simulink model "VCU_CS75_12_16_Test"  (R2014a)
settings: Solver=FixedStepDiscrete  StartTime=0.0  StopTime=25  FixedStep=0.0005  RelTol=1e-3
undefined symbols (not defined in the file): ecucoder_acal, I_SW01_L, LaterlAngleCommand, LDW, RemoteAcclPosition
libraries: simulink x913, ec5744lib x39
(part 23 of 30)

== system VCU_CS75_12_16_Test/长安CS75底盘程序，20ms一次/Output/Subsystem/TransmitMessages5/ACC_3F5/CRC ==
  CRC : Inport
  CRCRon : Rounding  Operator=round
  CRC_1sat : Saturate  UpperLimit=255  LowerLimit=0
  CRC_Convert : DataTypeConversion  OutDataTypeStr=uint8
  CRC_Convert1 : DataTypeConversion  OutDataTypeStr=uint32
  CRC_D : Product  Inputs=*/
  CRC_F : Constant  OutDataTypeStr=single
  CRC_L : simulink/Logic and Bit Operations/Bitwise Operator  logicop=AND  UseBitMask=on  BitMask=255  BitMaskRealWorld=Stored Integer
  CRC_O : Constant  Value=0  OutDataTypeStr=single
  CRC_S : ArithShift
  CRC_sat : Saturate  UpperLimit=0  LowerLimit=0
  CRC_st : Sum  Inputs=+-
  Constant{1..7} (7 alike) : Constant  Value=0  OutDataTypeStr=uint8
  output1 : Outport
  output2 : Outport  Port=2
  output3 : Outport  Port=3
  output4 : Outport  Port=4
  output5 : Outport  Port=5
  output6 : Outport  Port=6
  output7 : Outport  Port=7
  output8 : Outport  Port=8
  wires:
  CRC/1 -> CRC_sat/1
  CRC_sat/1 -> CRC_st/1
  CRC_O/1 -> CRC_st/2
  CRC_st/1 -> CRC_D/1
  CRC_F/1 -> CRC_D/2
  CRC_D/1 -> CRCRon/1
  CRCRon/1 -> CRC_S/1
  CRC_S/1 -> CRC_1sat/1
  CRC_1sat/1 -> CRC_Convert1/1
  CRC_Convert1/1 -> CRC_L/1
  CRC_L/1 -> CRC_Convert/1
  CRC_Convert/1 -> output8/1
  Constant1/1 -> output1/1
  Constant2/1 -> output2/1
  Constant3/1 -> output3/1
  Constant4/1 -> output4/1
  Constant5/1 -> output5/1
  Constant6/1 -> output6/1
  Constant7/1 -> output7/1

== system VCU_CS75_12_16_Test/长安CS75底盘程序，20ms一次/Output/Subsystem/TransmitMessages5/ACC_3F5/RollingConter ==
  RollingConter : Inport
  Constant{1..6,8} (7 alike) : Constant  Value=0  OutDataTypeStr=uint8
  RollingConterRon : Rounding  Operator=round
  RollingConter_1sat : Saturate  UpperLimit=15  LowerLimit=0
  RollingConter_Convert : DataTypeConversion  OutDataTypeStr=uint8
  RollingConter_Convert1 : DataTypeConversion  OutDataTypeStr=uint32
  RollingConter_D : Product  Inputs=*/
  RollingConter_F : Constant  OutDataTypeStr=single
  RollingConter_L : simulink/Logic and Bit Operations/Bitwise Operator  logicop=AND  UseBitMask=on  BitMask=15  BitMaskRealWorld=Stored Integer
  RollingConter_O : Constant  Value=0  OutDataTypeStr=single
  RollingConter_S : ArithShift
  RollingConter_sat : Saturate  UpperLimit=0  LowerLimit=0
  RollingConter_st : Sum  Inputs=+-
  output1 : Outport
  output2 : Outport  Port=2
  output3 : Outport  Port=3
  output4 : Outport  Port=4
  output5 : Outport  Port=5
  output6 : Outport  Port=6
  output7 : Outport  Port=7
  output8 : Outport  Port=8
  wires:
  RollingConter/1 -> RollingConter_sat/1
  RollingConter_sat/1 -> RollingConter_st/1
  RollingConter_O/1 -> RollingConter_st/2
  RollingConter_st/1 -> RollingConter_D/1
  RollingConter_F/1 -> RollingConter_D/2
  RollingConter_D/1 -> RollingConterRon/1
  RollingConterRon/1 -> RollingConter_S/1
  RollingConter_S/1 -> RollingConter_1sat/1
  RollingConter_1sat/1 -> RollingConter_Convert1/1
  RollingConter_Convert1/1 -> RollingConter_L/1
  RollingConter_L/1 -> RollingConter_Convert/1
  RollingConter_Convert/1 -> output7/1
  Constant1/1 -> output1/1
  Constant2/1 -> output2/1
  Constant3/1 -> output3/1
  Constant4/1 -> output4/1
  Constant5/1 -> output5/1
  Constant6/1 -> output6/1
  Constant8/1 -> output8/1

== system VCU_CS75_12_16_Test/长安CS75底盘程序，20ms一次/Output/Subsystem/TransmitMessages7/APA_29A/APA_ActivationStatus ==
  APA_ActivationStatus : Inport
  APA_ActivationStatusRon : Rounding  Operator=round
  APA_ActivationStatus_1sat : Saturate  UpperLimit=224  LowerLimit=0
  APA_ActivationStatus_Convert : DataTypeConversion  OutDataTypeStr=uint8
  APA_ActivationStatus_Convert1 : DataTypeConversion  OutDataTypeStr=uint32
  APA_ActivationStatus_D : Product  Inputs=*/
  APA_ActivationStatus_F : Constant  OutDataTypeStr=single
  APA_ActivationStatus_L : simulink/Logic and Bit Operations/Bitwise Operator  logicop=AND  UseBitMask=on  BitMask=224  BitMaskRealWorld=Stored Integer
  APA_ActivationStatus_O : Constant  Value=0  OutDataTypeStr=single
  APA_ActivationStatus_S : ArithShift  BitShiftNumber=-5
  APA_ActivationStatus_sat : Saturate  UpperLimit=7  LowerLimit=0
  APA_ActivationStatus_st : Sum  Inputs=+-
  Constant{1..5,7..8} (7 alike) : Constant  Value=0  OutDataTypeStr=uint8
  output1 : Outport
  output2 : Outport  Port=2
  output3 : Outport  Port=3
  output4 : Outport  Port=4
  output5 : Outport  Port=5
  output6 : Outport  Port=6
  output7 : Outport  Port=7
  output8 : Outport  Port=8
  wires:
  APA_ActivationStatus/1 -> APA_ActivationStatus_sat/1
  APA_ActivationStatus_sat/1 -> APA_ActivationStatus_st/1
  APA_ActivationStatus_O/1 -> APA_ActivationStatus_st/2
  APA_ActivationStatus_st/1 -> APA_ActivationStatus_D/1
  APA_ActivationStatus_F/1 -> APA_ActivationStatus_D/2
  APA_ActivationStatus_D/1 -> APA_ActivationStatusRon/1
  APA_ActivationStatusRon/1 -> APA_ActivationStatus_S/1
  APA_ActivationStatus_S/1 -> APA_ActivationStatus_1sat/1
  APA_ActivationStatus_1sat/1 -> APA_ActivationStatus_Convert1/1
  APA_ActivationStatus_Convert1/1 -> APA_ActivationStatus_L/1
  APA_ActivationStatus_L/1 -> APA_ActivationStatus_Convert/1
  APA_ActivationStatus_Convert/1 -> output6/1
  Constant1/1 -> output1/1
  Constant2/1 -> output2/1
  Constant3/1 -> output3/1
  Constant4/1 -> output4/1
  Constant5/1 -> output5/1
  Constant7/1 -> output7/1
  Constant8/1 -> output8/1

== system VCU_CS75_12_16_Test/长安CS75底盘程序，20ms一次/Output/Subsystem/TransmitMessages7/APA_29A/APA_Checksum ==
  APA_Checksum : Inport
  APA_ChecksumRon : Rounding  Operator=round
  APA_Checksum_1sat : Saturate  UpperLimit=240  LowerLimit=0
  APA_Checksum_Convert : DataTypeConversion  OutDataTypeStr=uint8
  APA_Checksum_Convert1 : DataTypeConversion  OutDataTypeStr=uint32
  APA_Checksum_D : Product  Inputs=*/
  APA_Checksum_F : Constant  OutDataTypeStr=single
  APA_Checksum_L : simulink/Logic and Bit Operations/Bitwise Operator  logicop=AND  UseBitMask=on  BitMask=240  BitMaskRealWorld=Stored Integer
  APA_Checksum_O : Constant  Value=0  OutDataTypeStr=single
  APA_Checksum_S : ArithShift  BitShiftNumber=-4
  APA_Checksum_sat : Saturate  UpperLimit=0  LowerLimit=0
  APA_Checksum_st : Sum  Inputs=+-
  Constant{1..7} (7 alike) : Constant  Value=0  OutDataTypeStr=uint8
  output1 : Outport
  output2 : Outport  Port=2
  output3 : Outport  Port=3
  output4 : Outport  Port=4
  output5 : Outport  Port=5
  output6 : Outport  Port=6
  output7 : Outport  Port=7
  output8 : Outport  Port=8
  wires:
  APA_Checksum/1 -> APA_Checksum_sat/1
  APA_Checksum_sat/1 -> APA_Checksum_st/1
  APA_Checksum_O/1 -> APA_Checksum_st/2
  APA_Checksum_st/1 -> APA_Checksum_D/1
  APA_Checksum_F/1 -> APA_Checksum_D/2
  APA_Checksum_D/1 -> APA_ChecksumRon/1
  APA_ChecksumRon/1 -> APA_Checksum_S/1
  APA_Checksum_S/1 -> APA_Checksum_1sat/1
  APA_Checksum_1sat/1 -> APA_Checksum_Convert1/1
  APA_Checksum_Convert1/1 -> APA_Checksum_L/1
  APA_Checksum_L/1 -> APA_Checksum_Convert/1
  APA_Checksum_Convert/1 -> output8/1
  Constant1/1 -> output1/1
  Constant2/1 -> output2/1
  Constant3/1 -> output3/1
  Constant4/1 -> output4/1
  Constant5/1 -> output5/1
  Constant6/1 -> output6/1
  Constant7/1 -> output7/1

== system VCU_CS75_12_16_Test/长安CS75底盘程序，20ms一次/Output/Subsystem/TransmitMessages7/APA_29A/APA_EPBrequest ==
  APA_EPBrequest : Inport
  APA_EPBrequestRon : Rounding  Operator=round
  APA_EPBrequest_1sat : Saturate  UpperLimit=3  LowerLimit=0
  APA_EPBrequest_Convert : DataTypeConversion  OutDataTypeStr=uint8
  APA_EPBrequest_Convert1 : DataTypeConversion  OutDataTypeStr=uint32
  APA_EPBrequest_D : Product  Inputs=*/
  APA_EPBrequest_F : Constant  OutDataTypeStr=single
  APA_EPBrequest_L : simulink/Logic and Bit Operations/Bitwise Operator  logicop=AND  UseBitMask=on  BitMask=3  BitMaskRealWorld=Stored Integer
  APA_EPBrequest_O : Constant  Value=0  OutDataTypeStr=single
  APA_EPBrequest_S : ArithShift
  APA_EPBrequest_sat : Saturate  UpperLimit=0  LowerLimit=0
  APA_EPBrequest_st : Sum  Inputs=+-
  Constant{2..8} (7 alike) : Constant  Value=0  OutDataTypeStr=uint8
  output1 : Outport
  output2 : Outport  Port=2
  output3 : Outport  Port=3
  output4 : Outport  Port=4
  output5 : Outport  Port=5
  output6 : Outport  Port=6
  output7 : Outport  Port=7
  output8 : Outport  Port=8
  wires:
  APA_EPBrequest/1 -> APA_EPBrequest_sat/1
  APA_EPBrequest_sat/1 -> APA_EPBrequest_st/1
  APA_EPBrequest_O/1 -> APA_EPBrequest_st/2
  APA_EPBrequest_st/1 -> APA_EPBrequest_D/1
  APA_EPBrequest_F/1 -> APA_EPBrequest_D/2
  APA_EPBrequest_D/1 -> APA_EPBrequestRon/1
  APA_EPBrequestRon/1 -> APA_EPBrequest_S/1
  APA_EPBrequest_S/1 -> APA_EPBrequest_1sat/1
  APA_EPBrequest_1sat/1 -> APA_EPBrequest_Convert1/1
  APA_EPBrequest_Convert1/1 -> APA_EPBrequest_L/1
  APA_EPBrequest_L/1 -> APA_EPBrequest_Convert/1
  APA_EPBrequest_Convert/1 -> output1/1
  Constant2/1 -> output2/1
  Constant3/1 -> output3/1
  Constant4/1 -> output4/1
  Constant5/1 -> output5/1
  Constant6/1 -> output6/1
  Constant7/1 -> output7/1
  Constant8/1 -> output8/1

== system VCU_CS75_12_16_Test/长安CS75底盘程序，20ms一次/Output/Subsystem/TransmitMessages7/APA_29A/APA_EPBrequestValid ==
  APA_EPBrequestValid : Inport
  APA_EPBrequestValidRon : Rounding  Operator=round
  APA_EPBrequestValid_1sat : Saturate  UpperLimit=4  LowerLimit=0
  APA_EPBrequestValid_Convert : DataTypeConversion  OutDataTypeStr=uint8
  APA_EPBrequestValid_Convert1 : DataTypeConversion  OutDataTypeStr=uint32
  APA_EPBrequestValid_D : Product  Inputs=*/
  APA_EPBrequestValid_F : Constant  OutDataTypeStr=single
  APA_EPBrequestValid_L : simulink/Logic and Bit Operations/Bitwise Operator  logicop=AND  UseBitMask=on  BitMask=4  BitMaskRealWorld=Stored Integer
  APA_EPBrequestValid_O : Constant  Value=0  OutDataTypeStr=single
  APA_EPBrequestValid_S : ArithShift  BitShiftNumber=-2
  APA_EPBrequestValid_sat : Saturate  UpperLimit=0  LowerLimit=0
  APA_EPBrequestValid_st : Sum  Inputs=+-
  Constant{2..8} (7 alike) : Constant  Value=0  OutDataTypeStr=uint8
  output1 : Outport
  output2 : Outport  Port=2
  output3 : Outport  Port=3
  output4 : Outport  Port=4
  output5 : Outport  Port=5
  output6 : Outport  Port=6
  output7 : Outport  Port=7
  output8 : Outport  Port=8
  wires:
  APA_EPBrequestValid/1 -> APA_EPBrequestValid_sat/1
  APA_EPBrequestValid_sat/1 -> APA_EPBrequestValid_st/1
  APA_EPBrequestValid_O/1 -> APA_EPBrequestValid_st/2
  APA_EPBrequestValid_st/1 -> APA_EPBrequestValid_D/1
  APA_EPBrequestValid_F/1 -> APA_EPBrequestValid_D/2
  APA_EPBrequestValid_D/1 -> APA_EPBrequestValidRon/1
  APA_EPBrequestValidRon/1 -> APA_EPBrequestValid_S/1
  APA_EPBrequestValid_S/1 -> APA_EPBrequestValid_1sat/1
  APA_EPBrequestValid_1sat/1 -> APA_EPBrequestValid_Convert1/1
  APA_EPBrequestValid_Convert1/1 -> APA_EPBrequestValid_L/1
  APA_EPBrequestValid_L/1 -> APA_EPBrequestValid_Convert/1
  APA_EPBrequestValid_Convert/1 -> output1/1
  Constant2/1 -> output2/1
  Constant3/1 -> output3/1
  Constant4/1 -> output4/1
  Constant5/1 -> output5/1
  Constant6/1 -> output6/1
  Constant7/1 -> output7/1
  Constant8/1 -> output8/1

== system VCU_CS75_12_16_Test/长安CS75底盘程序，20ms一次/Output/Subsystem/TransmitMessages7/APA_29A/APA_GearReqValid ==
  APA_GearReqValid : Inport
  APA_GearReqValidRon : Rounding  Operator=round
  APA_GearReqValid_1sat : Saturate  UpperLimit=4  LowerLimit=0
  APA_GearReqValid_Convert : DataTypeConversion  OutDataTypeStr=uint8
  APA_GearReqValid_Convert1 : DataTypeConversion  OutDataTypeStr=uint32
  APA_GearReqValid_D : Product  Inputs=*/
  APA_GearReqValid_F : Constant  OutDataTypeStr=single
  APA_GearReqValid_L : simulink/Logic and Bit Operations/Bitwise Operator  logicop=AND  UseBitMask=on  BitMask=4  BitMaskRealWorld=Stored Integer
  APA_GearReqValid_O : Constant  Value=0  OutDataTypeStr=single
  APA_GearReqValid_S : ArithShift  BitShiftNumber=-2
  APA_GearReqValid_sat : Saturate  UpperLimit=1  LowerLimit=0
  APA_GearReqValid_st : Sum  Inputs=+-
  Constant{1..3,5..8} (7 alike) : Constant  Value=0  OutDataTypeStr=uint8
  output1 : Outport
  output2 : Outport  Port=2
  output3 : Outport  Port=3
  output4 : Outport  Port=4
  output5 : Outport  Port=5
  output6 : Outport  Port=6
  output7 : Outport  Port=7
  output8 : Outport  Port=8
  wires:
  APA_GearReqValid/1 -> APA_GearReqValid_sat/1
  APA_GearReqValid_sat/1 -> APA_GearReqValid_st/1
  APA_GearReqValid_O/1 -> APA_GearReqValid_st/2
  APA_GearReqValid_st/1 -> APA_GearReqValid_D/1
  APA_GearReqValid_F/1 -> APA_GearReqValid_D/2
  APA_GearReqValid_D/1 -> APA_GearReqValidRon/1
  APA_GearReqValidRon/1 -> APA_GearReqValid_S/1
  APA_GearReqValid_S/1 -> APA_GearReqValid_1sat/1
  APA_GearReqValid_1sat/1 -> APA_GearReqValid_Convert1/1
  APA_GearReqValid_Convert1/1 -> APA_GearReqValid_L/1
  APA_GearReqValid_L/1 -> APA_GearReqValid_Convert/1
  APA_GearReqValid_Convert/1 -> output4/1
  Constant1/1 -> output1/1
  Constant2/1 -> output2/1
  Constant3/1 -> output3/1
  Constant5/1 -> output5/1
  Constant6/1 -> output6/1
  Constant7/1 -> output7/1
  Constant8/1 -> output8/1

== system VCU_CS75_12_16_Test/长安CS75底盘程序，20ms一次/Output/Subsystem/TransmitMessages7/APA_29A/APA_LSCAction ==
  APA_LSCAction : Inport
  APA_LSCActionRon : Rounding  Operator=round
  APA_LSCAction_1sat : Saturate  UpperLimit=8  LowerLimit=0
  APA_LSCAction_Convert : DataTypeConversion  OutDataTypeStr=uint8
  APA_LSCAction_Convert1 : DataTypeConversion  OutDataTypeStr=uint32
  APA_LSCAction_D : Product  Inputs=*/
  APA_LSCAction_F : Constant  OutDataTypeStr=single
  APA_LSCAction_L : simulink/Logic and Bit Operations/Bitwise Operator  logicop=AND  UseBitMask=on  BitMask=8  BitMaskRealWorld=Stored Integer
  APA_LSCAction_O : Constant  Value=0  OutDataTypeStr=single
  APA_LSCAction_S : ArithShift  BitShiftNumber=-3
  APA_LSCAction_sat : Saturate  UpperLimit=0  LowerLimit=0
  APA_LSCAction_st : Sum  Inputs=+-
  Constant{1..3,5..8} (7 alike) : Constant  Value=0  OutDataTypeStr=uint8
  output1 : Outport
  output2 : Outport  Port=2
  output3 : Outport  Port=3
  output4 : Outport  Port=4
  output5 : Outport  Port=5
  output6 : Outport  Port=6
  output7 : Outport  Port=7
  output8 : Outport  Port=8
  wires:
  APA_LSCAction/1 -> APA_LSCAction_sat/1
  APA_LSCAction_sat/1 -> APA_LSCAction_st/1
  APA_LSCAction_O/1 -> APA_LSCAction_st/2
  APA_LSCAction_st/1 -> APA_LSCAction_D/1
  APA_LSCAction_F/1 -> APA_LSCAction_D/2
  APA_LSCAction_D/1 -> APA_LSCActionRon/1
  APA_LSCActionRon/1 -> APA_LSCAction_S/1
  APA_LSCAction_S/1 -> APA_LSCAction_1sat/1
  APA_LSCAction_1sat/1 -> APA_LSCAction_Convert1/1
  APA_LSCAction_Convert1/1 -> APA_LSCAction_L/1
  APA_LSCAction_L/1 -> APA_LSCAction_Convert/1
  APA_LSCAction_Convert/1 -> output4/1
  Constant1/1 -> output1/1
  Constant2/1 -> output2/1
  Constant3/1 -> output3/1
  Constant5/1 -> output5/1
  Constant6/1 -> output6/1
  Constant7/1 -> output7/1
  Constant8/1 -> output8/1

== system VCU_CS75_12_16_Test/长安CS75底盘程序，20ms一次/Output/Subsystem/TransmitMessages7/APA_29A/APA_RollingCounter ==
  APA_RollingCounter : Inport
  APA_RollingCounterRon : Rounding  Operator=round
  APA_RollingCounter_1sat : Saturate  UpperLimit=15  LowerLimit=0
  APA_RollingCounter_Convert : DataTypeConversion  OutDataTypeStr=uint8
  APA_RollingCounter_Convert1 : DataTypeConversion  OutDataTypeStr=uint32
  APA_RollingCounter_D : Product  Inputs=*/
  APA_RollingCounter_F : Constant  OutDataTypeStr=single
  APA_RollingCounter_L : simulink/Logic and Bit Operations/Bitwise Operator  logicop=AND  UseBitMask=on  BitMask=15  BitMaskRealWorld=Stored Integer
  APA_RollingCounter_O : Constant  Value=0  OutDataTypeStr=single
  APA_RollingCounter_S : ArithShift
  APA_RollingCounter_sat : Saturate  UpperLimit=0  LowerLimit=0
  APA_RollingCounter_st : Sum  Inputs=+-
  Constant{1..7} (7 alike) : Constant  Value=0  OutDataTypeStr=uint8
  output1 : Outport
  output2 : Outport  Port=2
  output3 : Outport  Port=3
  output4 : Outport  Port=4
  output5 : Outport  Port=5
  output6 : Outport  Port=6
  output7 : Outport  Port=7
  output8 : Outport  Port=8
  wires:
  APA_RollingCounter/1 -> APA_RollingCounter_sat/1
  APA_RollingCounter_sat/1 -> APA_RollingCounter_st/1
  APA_RollingCounter_O/1 -> APA_RollingCounter_st/2
  APA_RollingCounter_st/1 -> APA_RollingCounter_D/1
  APA_RollingCounter_F/1 -> APA_RollingCounter_D/2
  APA_RollingCounter_D/1 -> APA_RollingCounterRon/1
  APA_RollingCounterRon/1 -> APA_RollingCounter_S/1
  APA_RollingCounter_S/1 -> APA_RollingCounter_1sat/1
  APA_RollingCounter_1sat/1 -> APA_RollingCounter_Convert1/1
  APA_RollingCounter_Convert1/1 -> APA_RollingCounter_L/1
  APA_RollingCounter_L/1 -> APA_RollingCounter_Convert/1
  APA_RollingCounter_Convert/1 -> output8/1
  Constant1/1 -> output1/1
  Constant2/1 -> output2/1
  Constant3/1 -> output3/1
  Constant4/1 -> output4/1
  Constant5/1 -> output5/1
  Constant6/1 -> output6/1
  Constant7/1 -> output7/1

== system VCU_CS75_12_16_Test/长安CS75底盘程序，20ms一次/Output/Subsystem/TransmitMessages7/APA_29A/APA_TargetAcceleration ==
  APA_TargetAcceleration : Inport
  APA_TargetAccelerationBitCov : DataTypeConversion  OutDataTypeStr=uint8
  APA_TargetAccelerationCOV : DataTypeConversion  OutDataTypeStr=uint8
  APA_TargetAccelerationRon : Rounding  Operator=round
  APA_TargetAcceleration_1sat : Saturate  UpperLimit=16320  LowerLimit=0
  APA_TargetAcceleration_And : simulink/Logic and Bit Operations/Bitwise Operator  logicop=AND  UseBitMask=off  NumInputPorts=2  BitMask=bin2dec('11011001')  BitMaskRealWorld=Stored Integer
  APA_TargetAcceleration_And_C : Constant  Value=255  OutDataTypeStr=uint32
  APA_TargetAcceleration_Convert : DataTypeConversion  OutDataTypeStr=uint32
  APA_TargetAcceleration_D : Product  Inputs=*/
  APA_TargetAcceleration_D1 : Product  Inputs=*/
  APA_TargetAcceleration_F : Constant  Value=0.05  OutDataTypeStr=single
  APA_TargetAcceleration_L : simulink/Logic and Bit Operations/Bitwise Operator  logicop=AND  UseBitMask=on  BitMask=16320  BitMaskRealWorld=Stored Integer
  APA_TargetAcceleration_O : Constant  Value=-5  OutDataTypeStr=single
  APA_TargetAcceleration_S : ArithShift  BitShiftNumber=-6
  APA_TargetAcceleration_sat : Saturate  UpperLimit=0  LowerLimit=0
  APA_TargetAcceleration_st : Sum  Inputs=+-
  APA_TargetAccelerationoutput2_C : Constant  Value=256
  Constant{1,4..8} (6 alike) : Constant  Value=0  OutDataTypeStr=uint8
  output1 : Outport
  output2 : Outport  Port=2
  output3 : Outport  Port=3
  output4 : Outport  Port=4
  output5 : Outport  Port=5
  output6 : Outport  Port=6
  output7 : Outport  Port=7
  output8 : Outport  Port=8
  wires:
  APA_TargetAcceleration/1 -> APA_TargetAcceleration_sat/1
  APA_TargetAcceleration_sat/1 -> APA_TargetAcceleration_st/1
  APA_TargetAcceleration_O/1 -> APA_TargetAcceleration_st/2
  APA_TargetAcceleration_st/1 -> APA_TargetAcceleration_D/1
  APA_TargetAcceleration_F/1 -> APA_TargetAcceleration_D/2
  APA_TargetAcceleration_D/1 -> APA_TargetAccelerationRon/1
  APA_TargetAccelerationRon/1 -> APA_TargetAcceleration_S/1
  APA_TargetAcceleration_S/1 -> APA_TargetAcceleration_1sat/1
  APA_TargetAcceleration_1sat/1 -> APA_TargetAcceleration_Convert/1
  APA_TargetAcceleration_Convert/1 -> APA_TargetAcceleration_L/1
  APA_TargetAcceleration_L/1 -> APA_TargetAcceleration_D1/1, APA_TargetAcceleration_And/1
  APA_TargetAccelerationoutput2_C/1 -> APA_TargetAcceleration_D1/2
  APA_TargetAcceleration_D1/1 -> APA_TargetAccelerationCOV/1
  APA_TargetAccelerationCOV/1 -> output2/1
  APA_TargetAcceleration_And_C/1 -> APA_TargetAcceleration_And/2
  APA_TargetAcceleration_And/1 -> APA_TargetAccelerationBitCov/1
  APA_TargetAccelerationBitCov/1 -> output3/1
  Constant1/1 -> output1/1
  Constant4/1 -> output4/1
  Constant5/1 -> output5/1
  Constant6/1 -> output6/1
  Constant7/1 -> output7/1
  Constant8/1 -> output8/1

== system VCU_CS75_12_16_Test/长安CS75底盘程序，20ms一次/Output/Subsystem/TransmitMessages7/APA_29A/APA_TargetAccelerationValid ==
  APA_TargetAccelerationValid : Inport
  APA_TargetAccelerationValidRon : Rounding  Operator=round
  APA_TargetAccelerationValid_1sat : Saturate  UpperLimit=64  LowerLimit=0
  APA_TargetAccelerationValid_Convert : DataTypeConversion  OutDataTypeStr=uint8
  APA_TargetAccelerationValid_Convert1 : DataTypeConversion  OutDataTypeStr=uint32
  APA_TargetAccelerationValid_D : Product  Inputs=*/
  APA_TargetAccelerationValid_F : Constant  OutDataTypeStr=single
  APA_TargetAccelerationValid_L : simulink/Logic and Bit Operations/Bitwise Operator  logicop=AND  UseBitMask=on  BitMask=64  BitMaskRealWorld=Stored Integer
  APA_TargetAccelerationValid_O : Constant  Value=0  OutDataTypeStr=single
  APA_TargetAccelerationValid_S : ArithShift  BitShiftNumber=-6
  APA_TargetAccelerationValid_sat : Saturate  UpperLimit=0  LowerLimit=0
  APA_TargetAccelerationValid_st : Sum  Inputs=+-
  Constant{1,3..8} (7 alike) : Constant  Value=0  OutDataTypeStr=uint8
  output1 : Outport
  output2 : Outport  Port=2
  output3 : Outport  Port=3
  output4 : Outport  Port=4
  output5 : Outport  Port=5
  output6 : Outport  Port=6
  output7 : Outport  Port=7
  output8 : Outport  Port=8
  wires:
  APA_TargetAccelerationValid/1 -> APA_TargetAccelerationValid_sat/1
  APA_TargetAccelerationValid_sat/1 -> APA_TargetAccelerationValid_st/1
  APA_TargetAccelerationValid_O/1 -> APA_TargetAccelerationValid_st/2
  APA_TargetAccelerationValid_st/1 -> APA_TargetAccelerationValid_D/1
  APA_TargetAccelerationValid_F/1 -> APA_TargetAccelerationValid_D/2
  APA_TargetAccelerationValid_D/1 -> APA_TargetAccelerationValidRon/1
  APA_TargetAccelerationValidRon/1 -> APA_TargetAccelerationValid_S/1
  APA_TargetAccelerationValid_S/1 -> APA_TargetAccelerationValid_1sat/1
  APA_TargetAccelerationValid_1sat/1 -> APA_TargetAccelerationValid_Convert1/1
  APA_TargetAccelerationValid_Convert1/1 -> APA_TargetAccelerationValid_L/1
  APA_TargetAccelerationValid_L/1 -> APA_TargetAccelerationValid_Convert/1
  APA_TargetAccelerationValid_Convert/1 -> output2/1
  Constant1/1 -> output1/1
  Constant3/1 -> output3/1
  Constant4/1 -> output4/1
  Constant5/1 -> output5/1
  Constant6/1 -> output6/1
  Constant7/1 -> output7/1
  Constant8/1 -> output8/1

== system VCU_CS75_12_16_Test/长安CS75底盘程序，20ms一次/Output/Subsystem/TransmitMessages7/APA_29A/APA_TranShiftReqValid ==
  APA_TranShiftReqValid : Inport
  APA_TranShiftReqValidRon : Rounding  Operator=round
  APA_TranShiftReqValid_1sat : Saturate  UpperLimit=8  LowerLimit=0
  APA_TranShiftReqValid_Convert : DataTypeConversion  OutDataTypeStr=uint8
  APA_TranShiftReqValid_Convert1 : DataTypeConversion  OutDataTypeStr=uint32
  APA_TranShiftReqValid_D : Product  Inputs=*/
  APA_TranShiftReqValid_F : Constant  OutDataTypeStr=single
  APA_TranShiftReqValid_L : simulink/Logic and Bit Operations/Bitwise Operator  logicop=AND  UseBitMask=on  BitMask=8  BitMaskRealWorld=Stored Integer
  APA_TranShiftReqValid_O : Constant  Value=0  OutDataTypeStr=single
  APA_TranShiftReqValid_S : ArithShift  BitShiftNumber=-3
  APA_TranShiftReqValid_sat : Saturate  UpperLimit=1  LowerLimit=0
  APA_TranShiftReqValid_st : Sum  Inputs=+-
  Constant{2..8} (7 alike) : Constant  Value=0  OutDataTypeStr=uint8
  output1 : Outport
  output2 : Outport  Port=2
  output3 : Outport  Port=3
  output4 : Outport  Port=4
  output5 : Outport  Port=5
  output6 : Outport  Port=6
  output7 : Outport  Port=7
  output8 : Outport  Port=8
  wires:
  APA_TranShiftReqValid/1 -> APA_TranShiftReqValid_sat/1
  APA_TranShiftReqValid_sat/1 -> APA_TranShiftReqValid_st/1
  APA_TranShiftReqValid_O/1 -> APA_TranShiftReqValid_st/2
  APA_TranShiftReqValid_st/1 -> APA_TranShiftReqValid_D/1
  APA_TranShiftReqValid_F/1 -> APA_TranShiftReqValid_D/2
  APA_TranShiftReqValid_D/1 -> APA_TranShiftReqValidRon/1
  APA_TranShiftReqValidRon/1 -> APA_TranShiftReqValid_S/1
  APA_TranShiftReqValid_S/1 -> APA_TranShiftReqValid_1sat/1
  APA_TranShiftReqValid_1sat/1 -> APA_TranShiftReqValid_Convert1/1
  APA_TranShiftReqValid_Convert1/1 -> APA_TranShiftReqValid_L/1
  APA_TranShiftReqValid_L/1 -> APA_TranShiftReqValid_Convert/1
  APA_TranShiftReqValid_Convert/1 -> output1/1
  Constant2/1 -> output2/1
  Constant3/1 -> output3/1
  Constant4/1 -> output4/1
  Constant5/1 -> output5/1
  Constant6/1 -> output6/1
  Constant7/1 -> output7/1
  Constant8/1 -> output8/1

== system VCU_CS75_12_16_Test/长安CS75底盘程序，20ms一次/Output/Subsystem/TransmitMessages7/APA_29A/APA_TranShiftRequest ==
  APA_TranShiftRequest : Inport
  APA_TranShiftRequestRon : Rounding  Operator=round
  APA_TranShiftRequest_1sat : Saturate  UpperLimit=112  LowerLimit=0
  APA_TranShiftRequest_Convert : DataTypeConversion  OutDataTypeStr=uint8
  APA_TranShiftRequest_Convert1 : DataTypeConversion  OutDataTypeStr=uint32
  APA_TranShiftRequest_D : Product  Inputs=*/
  APA_TranShiftRequest_F : Constant  OutDataTypeStr=single
  APA_TranShiftRequest_L : simulink/Logic and Bit Operations/Bitwise Operator  logicop=AND  UseBitMask=on  BitMask=112  BitMaskRealWorld=Stored Integer
  APA_TranShiftRequest_O : Constant  Value=0  OutDataTypeStr=single
  APA_TranShiftRequest_S : ArithShift  BitShiftNumber=-4
  APA_TranShiftRequest_sat : Saturate  UpperLimit=7  LowerLimit=0
  APA_TranShiftRequest_st : Sum  Inputs=+-
  Constant{2..8} (7 alike) : Constant  Value=0  OutDataTypeStr=uint8
  output1 : Outport
  output2 : Outport  Port=2
  output3 : Outport  Port=3
  output4 : Outport  Port=4
  output5 : Outport  Port=5
  output6 : Outport  Port=6
  output7 : Outport  Port=7
  output8 : Outport  Port=8
  wires:
  APA_TranShiftRequest/1 -> APA_TranShiftRequest_sat/1
  APA_TranShiftRequest_sat/1 -> APA_TranShiftRequest_st/1
  APA_TranShiftRequest_O/1 -> APA_TranShiftRequest_st/2
  APA_TranShiftRequest_st/1 -> APA_TranShiftRequest_D/1
  APA_TranShiftRequest_F/1 -> APA_TranShiftRequest_D/2
  APA_TranShiftRequest_D/1 -> APA_TranShiftRequestRon/1
  APA_TranShiftRequestRon/1 -> APA_TranShiftRequest_S/1
  APA_TranShiftRequest_S/1 -> APA_TranShiftRequest_1sat/1
  APA_TranShiftRequest_1sat/1 -> APA_TranShiftRequest_Convert1/1
  APA_TranShiftRequest_Convert1/1 -> APA_TranShiftRequest_L/1
  APA_TranShiftRequest_L/1 -> APA_TranShiftRequest_Convert/1
  APA_TranShiftRequest_Convert/1 -> output1/1
  Constant2/1 -> output2/1
  Constant3/1 -> output3/1
  Constant4/1 -> output4/1
  Constant5/1 -> output5/1
  Constant6/1 -> output6/1
  Constant7/1 -> output7/1
  Constant8/1 -> output8/1

== system VCU_CS75_12_16_Test/长安CS75底盘程序，20ms一次/Output/Subsystem/TransmitMessages8/APA_2D4/APA_APAStatus ==
  APA_APAStatus : Inport
  APA_APAStatusRon : Rounding  Operator=round
  APA_APAStatus_1sat : Saturate  UpperLimit=127  LowerLimit=0
  APA_APAStatus_Convert : DataTypeConversion  OutDataTypeStr=uint8
  APA_APAStatus_Convert1 : DataTypeConversion  OutDataTypeStr=uint32
  APA_APAStatus_D : Product  Inputs=*/
  APA_APAStatus_F : Constant  OutDataTypeStr=single
  APA_APAStatus_L : simulink/Logic and Bit Operations/Bitwise Operator  logicop=AND  UseBitMask=on  BitMask=127  BitMaskRealWorld=Stored Integer
  APA_APAStatus_O : Constant  Value=0  OutDataTypeStr=single
  APA_APAStatus_S : ArithShift
  APA_APAStatus_sat : Saturate  UpperLimit=127  LowerLimit=0
  APA_APAStatus_st : Sum  Inputs=+-
  Constant{2..8} (7 alike) : Constant  Value=0  OutDataTypeStr=uint8
  output1 : Outport
  output2 : Outport  Port=2
  output3 : Outport  Port=3
  output4 : Outport  Port=4
  output5 : Outport  Port=5
  output6 : Outport  Port=6
  output7 : Outport  Port=7
  output8 : Outport  Port=8
  wires:
  APA_APAStatus/1 -> APA_APAStatus_sat/1
  APA_APAStatus_sat/1 -> APA_APAStatus_st/1
  APA_APAStatus_O/1 -> APA_APAStatus_st/2
  APA_APAStatus_st/1 -> APA_APAStatus_D/1
  APA_APAStatus_F/1 -> APA_APAStatus_D/2
  APA_APAStatus_D/1 -> APA_APAStatusRon/1
  APA_APAStatusRon/1 -> APA_APAStatus_S/1
  APA_APAStatus_S/1 -> APA_APAStatus_1sat/1
  APA_APAStatus_1sat/1 -> APA_APAStatus_Convert1/1
  APA_APAStatus_Convert1/1 -> APA_APAStatus_L/1
  APA_APAStatus_L/1 -> APA_APAStatus_Convert/1
  APA_APAStatus_Convert/1 -> output1/1
  Constant2/1 -> output2/1
  Constant3/1 -> output3/1
  Constant4/1 -> output4/1
  Constant5/1 -> output5/1
  Constant6/1 -> output6/1
  Constant7/1 -> output7/1
  Constant8/1 -> output8/1

== system VCU_CS75_12_16_Test/长安CS75底盘程序，20ms一次/Output/Subsystem/TransmitMessages8/APA_2D4/APA_ReleasePressureReq ==
  APA_ReleasePressureReq : Inport
  APA_ReleasePressureReqRon : Rounding  Operator=round
  APA_ReleasePressureReq_1sat : Saturate  UpperLimit=16  LowerLimit=0
  APA_ReleasePressureReq_Convert : DataTypeConversion  OutDataTypeStr=uint8
  APA_ReleasePressureReq_Convert1 : DataTypeConversion  OutDataTypeStr=uint32
  APA_ReleasePressureReq_D : Product  Inputs=*/
  APA_ReleasePressureReq_F : Constant  OutDataTypeStr=single
  APA_ReleasePressureReq_L : simulink/Logic and Bit Operations/Bitwise Operator  logicop=AND  UseBitMask=on  BitMask=16  BitMaskRealWorld=Stored Integer
  APA_ReleasePressureReq_O : Constant  Value=0  OutDataTypeStr=single
  APA_ReleasePressureReq_S : ArithShift  BitShiftNumber=-4
  APA_ReleasePressureReq_sat : Saturate  UpperLimit=1  LowerLimit=0
  APA_ReleasePressureReq_st : Sum  Inputs=+-
  Constant{1..4,6..8} (7 alike) : Constant  Value=0  OutDataTypeStr=uint8
  output1 : Outport
  output2 : Outport  Port=2
  output3 : Outport  Port=3
  output4 : Outport  Port=4
  output5 : Outport  Port=5
  output6 : Outport  Port=6
  output7 : Outport  Port=7
  output8 : Outport  Port=8
  wires:
  APA_ReleasePressureReq/1 -> APA_ReleasePressureReq_sat/1
  APA_ReleasePressureReq_sat/1 -> APA_ReleasePressureReq_st/1
  APA_ReleasePressureReq_O/1 -> APA_ReleasePressureReq_st/2
  APA_ReleasePressureReq_st/1 -> APA_ReleasePressureReq_D/1
  APA_ReleasePressureReq_F/1 -> APA_ReleasePressureReq_D/2
  APA_ReleasePressureReq_D/1 -> APA_ReleasePressureReqRon/1
  APA_ReleasePressureReqRon/1 -> APA_ReleasePressureReq_S/1
  APA_ReleasePressureReq_S/1 -> APA_ReleasePressureReq_1sat/1
  APA_ReleasePressureReq_1sat/1 -> APA_ReleasePressureReq_Convert1/1
  APA_ReleasePressureReq_Convert1/1 -> APA_ReleasePressureReq_L/1
  APA_ReleasePressureReq_L/1 -> APA_ReleasePressureReq_Convert/1
  APA_ReleasePressureReq_Convert/1 -> output5/1
  Constant1/1 -> output1/1
  Constant2/1 -> output2/1
  Constant3/1 -> output3/1
  Constant4/1 -> output4/1
  Constant6/1 -> output6/1
  Constant7/1 -> output7/1
  Constant8/1 -> output8/1

== system VCU_CS75_12_16_Test/长安CS75底盘程序，20ms一次/Output/Subsystem/TransmitMessages8/APA_2D4/CRC ==
  CRC : Inport
  CRCRon : Rounding  Operator=round
  CRC_1sat : Saturate  UpperLimit=255  LowerLimit=0
  CRC_Convert : DataTypeConversion  OutDataTypeStr=uint8
  CRC_Convert1 : DataTypeConversion  OutDataTypeStr=uint32
  CRC_D : Product  Inputs=*/
  CRC_F : Constant  OutDataTypeStr=single
  CRC_L : simulink/Logic and Bit Operations/Bitwise Operator  logicop=AND  UseBitMask=on  BitMask=255  BitMaskRealWorld=Stored Integer
  CRC_O : Constant  Value=0  OutDataTypeStr=single
  CRC_S : ArithShift
  CRC_sat : Saturate  UpperLimit=0  LowerLimit=0
  CRC_st : Sum  Inputs=+-
  Constant{1..7} (7 alike) : Constant  Value=0  OutDataTypeStr=uint8
  output1 : Outport
  output2 : Outport  Port=2
  output3 : Outport  Port=3
  output4 : Outport  Port=4
  output5 : Outport  Port=5
  output6 : Outport  Port=6
  output7 : Outport  Port=7
  output8 : Outport  Port=8
  wires:
  CRC/1 -> CRC_sat/1
  CRC_sat/1 -> CRC_st/1
  CRC_O/1 -> CRC_st/2
  CRC_st/1 -> CRC_D/1
  CRC_F/1 -> CRC_D/2
  CRC_D/1 -> CRCRon/1
  CRCRon/1 -> CRC_S/1
  CRC_S/1 -> CRC_1sat/1
  CRC_1sat/1 -> CRC_Convert1/1
  CRC_Convert1/1 -> CRC_L/1
  CRC_L/1 -> CRC_Convert/1
  CRC_Convert/1 -> output8/1
  Constant1/1 -> output1/1
  Constant2/1 -> output2/1
  Constant3/1 -> output3/1
  Constant4/1 -> output4/1
  Constant5/1 -> output5/1
  Constant6/1 -> output6/1
  Constant7/1 -> output7/1

== system VCU_CS75_12_16_Test/长安CS75底盘程序，20ms一次/Output/Subsystem/TransmitMessages8/APA_2D4/RollingConter ==
  RollingConter : Inport
  Constant{1..6,8} (7 alike) : Constant  Value=0  OutDataTypeStr=uint8
  RollingConterRon : Rounding  Operator=round
  RollingConter_1sat : Saturate  UpperLimit=15  LowerLimit=0
  RollingConter_Convert : DataTypeConversion  OutDataTypeStr=uint8
  RollingConter_Convert1 : DataTypeConversion  OutDataTypeStr=uint32
  RollingConter_D : Product  Inputs=*/
  RollingConter_F : Constant  OutDataTypeStr=single
  RollingConter_L : simulink/Logic and Bit Operations/Bitwise Operator  logicop=AND  UseBitMask=on  BitMask=15  BitMaskRealWorld=Stored Integer
  RollingConter_O : Constant  Value=0  OutDataTypeStr=single
  RollingConter_S : ArithShift
  RollingConter_sat : Saturate  UpperLimit=0  LowerLimit=0
  RollingConter_st : Sum  Inputs=+-
  output1 : Outport
  output2 : Outport  Port=2
  output3 : Outport  Port=3
  output4 : Outport  Port=4
  output5 : Outport  Port=5
  output6 : Outport  Port=6
  output7 : Outport  Port=7
  output8 : Outport  Port=8
  wires:
  RollingConter/1 -> RollingConter_sat/1
  RollingConter_sat/1 -> RollingConter_st/1
  RollingConter_O/1 -> RollingConter_st/2
  RollingConter_st/1 -> RollingConter_D/1
  RollingConter_F/1 -> RollingConter_D/2
  RollingConter_D/1 -> RollingConterRon/1
  RollingConterRon/1 -> RollingConter_S/1
  RollingConter_S/1 -> RollingConter_1sat/1
  RollingConter_1sat/1 -> RollingConter_Convert1/1
  RollingConter_Convert1/1 -> RollingConter_L/1
  RollingConter_L/1 -> RollingConter_Convert/1
  RollingConter_Convert/1 -> output7/1
  Constant1/1 -> output1/1
  Constant2/1 -> output2/1
  Constant3/1 -> output3/1
  Constant4/1 -> output4/1
  Constant5/1 -> output5/1
  Constant6/1 -> output6/1
  Constant8/1 -> output8/1

== system VCU_CS75_12_16_Test/长安CS75底盘程序，20ms一次/Input/CAN0_Rx/a1_211/ReceiveMessages/Subsystem/a1 ==
  input : Inport
  Demux : Demux  Outputs=8
  SCS_Ad : Sum
  SCS_Convert : DataTypeConversion  OutDataTypeStr=uint32
  SCS_F : Gain
  SCS_L : simulink/Logic and Bit Operations/Bitwise Operator  logicop=AND  UseBitMask=on  BitMask=8  BitMaskRealWorld=Stored Integer
  SCS_O : Constant  Value=0  OutDataTypeStr=single
  SCS_S : ArithShift  BitShiftNumber=3
  SCS_Sub : Subsystem
  SCS_sat : Saturate  UpperLimit=1  LowerLimit=0
  SCScv : DataTypeConversion
  Vx_Ad : Sum
  Vx_Convert : DataTypeConversion  OutDataTypeStr=uint32
  Vx_F : Gain  Gain=0.00610360875867857
  Vx_L : simulink/Logic and Bit Operations/Bitwise Operator  logicop=AND  UseBitMask=on  BitMask=65535  BitMaskRealWorld=Stored Integer
  Vx_O : Constant  Value=-200  OutDataTypeStr=single
  Vx_S : ArithShift
  Vx_Sub : Subsystem
  Vx_sat : Saturate  UpperLimit=200  LowerLimit=-200
  Vxcv : DataTypeConversion
  Vxinput8_Ad : Sum
  Vxinput8_C : Constant  Value=256
  Vxinput8_P : Product
  cones_count_actual_Ad : Sum
  cones_count_actual_Convert : DataTypeConversion  OutDataTypeStr=uint32
  cones_count_actual_F : Gain
  cones_count_actual_L : simulink/Logic and Bit Operations/Bitwise Operator  logicop=AND  UseBitMask=on  BitMask=255  BitMaskRealWorld=Stored Integer
  cones_count_actual_O : Constant  Value=0  OutDataTypeStr=single
  cones_count_actual_S : ArithShift
  cones_count_actual_Sub : Subsystem
  cones_count_actual_sat : Saturate  UpperLimit=255  LowerLimit=0
  cones_count_actualcv : DataTypeConversion
  cones_count_all_Ad : Sum
  cones_count_all_Convert : DataTypeConversion  OutDataTypeStr=uint32
  cones_count_all_F : Gain
  cones_count_all_L : simulink/Logic and Bit Operations/Bitwise Operator  logicop=AND  UseBitMask=on  BitMask=255  BitMaskRealWorld=Stored Integer
  cones_count_all_O : Constant  Value=0  OutDataTypeStr=single
  cones_count_all_S : ArithShift
  cones_count_all_Sub : Subsystem
  cones_count_all_sat : Saturate  UpperLimit=255  LowerLimit=0
  cones_count_allcv : DataTypeConversion
  finish_Ad : Sum
  finish_Convert : DataTypeConversion  OutDataTypeStr=uint32
  finish_F : Gain
  finish_L : simulink/Logic and Bit Operations/Bitwise Operator  logicop=AND  UseBitMask=on  BitMask=4  BitMaskRealWorld=Stored Integer
  finish_O : Constant  Value=0  OutDataTypeStr=single
  finish_S : ArithShift  BitShiftNumber=2
  finish_Sub : Subsystem
  finish_sat : Saturate  UpperLimit=1  LowerLimit=0
  finishcv : DataTypeConversion
  mission_Ad : Sum
  mission_Convert : DataTypeConversion  OutDataTypeStr=uint32
  mission_F : Gain
  mission_L : simulink/Logic and Bit Operations/Bitwise Operator  logicop=AND  UseBitMask=on  BitMask=240  BitMaskRealWorld=Stored Integer
  mission_O : Constant  Value=0  OutDataTypeStr=single
  mission_S : ArithShift  BitShiftNumber=4
  mission_Sub : Subsystem
  mission_sat : Saturate  UpperLimit=7  LowerLimit=0
  missioncv : DataTypeConversion
  tap_Ad : Sum
  tap_Convert : DataTypeConversion  OutDataTypeStr=uint32
  tap_F : Gain
  tap_L : simulink/Logic and Bit Operations/Bitwise Operator  logicop=AND  UseBitMask=on  BitMask=3  BitMaskRealWorld=Stored Integer
  tap_O : Constant  Value=0  OutDataTypeStr=single
  tap_S : ArithShift
  tap_Sub : Subsystem
  tap_sat : Saturate  UpperLimit=3  LowerLimit=0
  tapcv : DataTypeConversion
  target_steering_Ad : Sum
  target_steering_Convert : DataTypeConversion  OutDataTypeStr=uint32
  target_steering_F : Gain  Gain=0.0488400488400488
  target_steering_L : simulink/Logic and Bit Operations/Bitwise Operator  logicop=AND  UseBitMask=on  BitMask=4095  BitMaskRealWorld=Stored Integer
  target_steering_O : Constant  Value=-100  OutDataTypeStr=single
  target_steering_S : ArithShift
  target_steering_Sub : Subsystem
  target_steering_sat : Saturate  UpperLimit=99.9999999999998  LowerLimit=-100
  target_steeringcv : DataTypeConversion
  target_steeringinput2_Ad : Sum
  target_steeringinput2_C : Constant  Value=256
  target_steeringinput2_P : Product
  throttlevbrake_position_Ad : Sum
  throttlevbrake_position_Convert : DataTypeConversion  OutDataTypeStr=uint32
  throttlevbrake_position_F : Gain  Gain=0.0488400488400488
  throttlevbrake_position_L : simulink/Logic and Bit Operations/Bitwise Operator  logicop=AND  UseBitMask=on  BitMask=65520  BitMaskRealWorld=Stored Integer
  throttlevbrake_position_O : Constant  Value=-100  OutDataTypeStr=single
  throttlevbrake_position_S : ArithShift  BitShiftNumber=4
  throttlevbrake_position_Sub : Subsystem
  throttlevbrake_position_sat : Saturate  UpperLimit=100  LowerLimit=-100
  throttlevbrake_positioncv : DataTypeConversion
  throttlevbrake_positioninput3_Ad : Sum
  throttlevbrake_positioninput3_C : Constant  Value=256
  throttlevbrake_positioninput3_P : Product
  Vx_Out : Outport
  mission_Out : Outport  Port=2
  SCS_Out : Outport  Port=3
  finish_Out : Outport  Port=4
  tap_Out : Outport  Port=5
  cones_count_all_Out : Outport  Port=6
  cones_count_actual_Out : Outport  Port=7
  throttlevbrake_position_Out : Outport  Port=8
  target_steering_Out : Outport  Port=9
  wires:
  Vx_F/1 -> Vx_Ad/1
  Vx_O/1 -> Vx_Ad/2
  Vx_Ad/1 -> Vx_sat/1
  Vx_sat/1 -> Vx_Out/1
  Demux/8 -> Vxinput8_P/1
  Vxinput8_C/1 -> Vxinput8_P/2
  Vxinput8_P/1 -> Vxinput8_Ad/1
  Demux/7 -> Vxinput8_Ad/2
  Vxinput8_Ad/1 -> Vx_Sub/1(In1)
  Vx_Sub/1(Out1) -> Vx_Convert/1
  Vx_Convert/1 -> Vx_L/1
  Vx_L/1 -> Vx_S/1
  Vx_S/1 -> Vxcv/1
  Vxcv/1 -> Vx_F/1
  mission_F/1 -> mission_Ad/1
  mission_O/1 -> mission_Ad/2
  mission_Ad/1 -> mission_sat/1
  mission_sat/1 -> mission_Out/1
  Demux/6 -> mission_Sub/1(In1), SCS_Sub/1(In1), finish_Sub/1(In1), tap_Sub/1(In1)
  mission_Sub/1(Out1) -> mission_Convert/1
  mission_Convert/1 -> mission_L/1
  mission_L/1 -> mission_S/1
  mission_S/1 -> missioncv/1
  missioncv/1 -> mission_F/1
  SCS_F/1 -> SCS_Ad/1
  SCS_O/1 -> SCS_Ad/2
  SCS_Ad/1 -> SCS_sat/1
  SCS_sat/1 -> SCS_Out/1
  SCS_Sub/1(Out1) -> SCS_Convert/1
  SCS_Convert/1 -> SCS_L/1
  SCS_L/1 -> SCS_S/1
  SCS_S/1 -> SCScv/1
  SCScv/1 -> SCS_F/1
  finish_F/1 -> finish_Ad/1
  finish_O/1 -> finish_Ad/2
  finish_Ad/1 -> finish_sat/1
  finish_sat/1 -> finish_Out/1
  finish_Sub/1(Out1) -> finish_Convert/1
  finish_Convert/1 -> finish_L/1
  finish_L/1 -> finish_S/1
  finish_S/1 -> finishcv/1
  finishcv/1 -> finish_F/1
  tap_F/1 -> tap_Ad/1
  tap_O/1 -> tap_Ad/2
  tap_Ad/1 -> tap_sat/1
  tap_sat/1 -> tap_Out/1
  tap_Sub/1(Out1) -> tap_Convert/1
  tap_Convert/1 -> tap_L/1
  tap_L/1 -> tap_S/1
  tap_S/1 -> tapcv/1
  tapcv/1 -> tap_F/1
  cones_count_all_F/1 -> cones_count_all_Ad/1
  cones_count_all_O/1 -> cones_count_all_Ad/2
  cones_count_all_Ad/1 -> cones_count_all_sat/1
  cones_count_all_sat/1 -> cones_count_all_Out/1
  Demux/5 -> cones_count_all_Sub/1(In1)
  cones_count_all_Sub/1(Out1) -> cones_count_all_Convert/1
  cones_count_all_Convert/1 -> cones_count_all_L/1
  cones_count_all_L/1 -> cones_count_all_S/1
  cones_count_all_S/1 -> cones_count_allcv/1
  cones_count_allcv/1 -> cones_count_all_F/1
  cones_count_actual_F/1 -> cones_count_actual_Ad/1
  cones_count_actual_O/1 -> cones_count_actual_Ad/2
  cones_count_actual_Ad/1 -> cones_count_actual_sat/1
  cones_count_actual_sat/1 -> cones_count_actual_Out/1
  Demux/4 -> cones_count_actual_Sub/1(In1)
  cones_count_actual_Sub/1(Out1) -> cones_count_actual_Convert/1
  cones_count_actual_Convert/1 -> cones_count_actual_L/1
  cones_count_actual_L/1 -> cones_count_actual_S/1
  cones_count_actual_S/1 -> cones_count_actualcv/1
  cones_count_actualcv/1 -> cones_count_actual_F/1
  throttlevbrake_position_F/1 -> throttlevbrake_position_Ad/1
  throttlevbrake_position_O/1 -> throttlevbrake_position_Ad/2
  throttlevbrake_position_Ad/1 -> throttlevbrake_position_sat/1
  throttlevbrake_position_sat/1 -> throttlevbrake_position_Out/1
  Demux/3 -> throttlevbrake_positioninput3_P/1
  throttlevbrake_positioninput3_C/1 -> throttlevbrake_positioninput3_P/2
  throttlevbrake_positioninput3_P/1 -> throttlevbrake_positioninput3_Ad/1
  Demux/2 -> throttlevbrake_positioninput3_Ad/2, target_steeringinput2_P/1
  throttlevbrake_positioninput3_Ad/1 -> throttlevbrake_position_Sub/1(In1)
  throttlevbrake_position_Sub/1(Out1) -> throttlevbrake_position_Convert/1
  throttlevbrake_position_Convert/1 -> throttlevbrake_position_L/1
  throttlevbrake_position_L/1 -> throttlevbrake_position_S/1
  throttlevbrake_position_S/1 -> throttlevbrake_positioncv/1
  throttlevbrake_positioncv/1 -> throttlevbrake_position_F/1
  target_steering_F/1 -> target_steering_Ad/1
  target_steering_O/1 -> target_steering_Ad/2
  target_steering_Ad/1 -> target_steering_sat/1
  target_steering_sat/1 -> target_steering_Out/1
  target_steeringinput2_C/1 -> target_steeringinput2_P/2
  target_steeringinput2_P/1 -> target_steeringinput2_Ad/1
  Demux/1 -> target_steeringinput2_Ad/2
  target_steeringinput2_Ad/1 -> target_steering_Sub/1(In1)
  target_steering_Sub/1(Out1) -> target_steering_Convert/1
  target_steering_Convert/1 -> target_steering_L/1
  target_steering_L/1 -> target_steering_S/1
  target_steering_S/1 -> target_steeringcv/1
  target_steeringcv/1 -> target_steering_F/1
  input/1 -> Demux/1
